simulink library "VLSGen"  (R2022b)
settings: Solver=VariableStepAuto  StartTime=0.0  StopTime=10.0  RelTol=1e-3
undefined symbols (not defined in the file or in its folder): Row, VLSConfig
libraries: TuneVar x3, TOP x2, FirGenericDeprecated x1, FeaturePath x1, FirGeneric x1
settings Model: Creator=ud1041536  LastModifiedBy=mt1047270
settings SolverCC: AlgebraicLoopSolver=TrustRegion
settings DataIOCC: ReturnWorkspaceOutputs=off
settings DebuggingCC: UnconnectedInputMsg=warning  UnconnectedOutputMsg=warning  UnconnectedLineMsg=warning  SFMachineParentedDataDiag=warning  ArithmeticOperatorsInVariantConditions=warning
settings ModelReferenceCC: EnableRefExpFcnMdlSchedulingChecks=on
settings SFSimCC: CustomCodeUndefinedFunction=UseInterfaceOnly

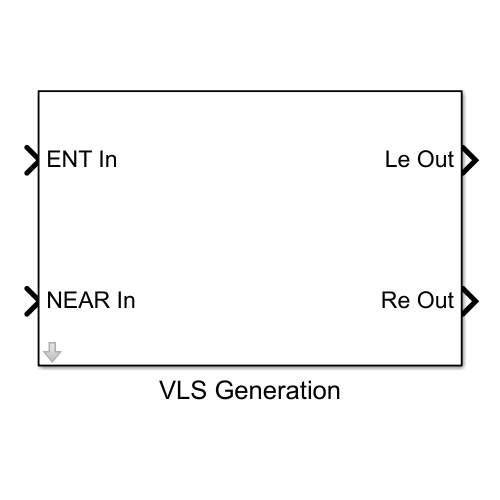
[thumbnail: Simulink's stored preview of the top-level diagram]
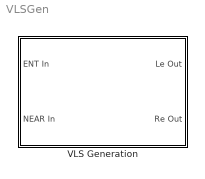
== system VLSGen ==
  VLS Generation : Subsystem  mask{configStruct=VLSConfig.VLSGenConfig, FeatureName=Generation}
      mask prompts: configStruct "Config struct name:"; FeatureName "Feature path name:"
      mask init:
      | % Get block parameters from configStruct
      | variantFIR = configStruct.variantFIR;
      | frameSize = configStruct.frameSize;
      | numFilters = configStruct.numFilters;
      | maxTotalFirLength = configStruct.maxTotalFirLength;
      | 
      | % Get block default values
      | firCoeffsDefault = configStruct.firCoeffsDefault;
      | firLengthsDefault = configStruct.firLengthsDefault;
      | 
      | % Set implementation type for FIR
      | % firBlockPath = MaskUtil.SubBlockName(gcbh, 'FIR');
      | % firBlockHandle = getSimulinkBlockHandle(firBlockPath);
      | % if -1 ~= firBlockHandle
      | %     set_param(firBlockHandle, 'variantSelect', variantFIR);
      | %     if variantFIR == 1 % Set two extras block params for Accel implementation
      | %         set_param(firBlockHandle, 'numIn', num2str(4));
      | %         set_param(firBlockHandle, 'frameSize', num2str(frameSize));
      | %     end
      | % end
      mask TypeOptions FeatureName: FeaturePath/FeatureName

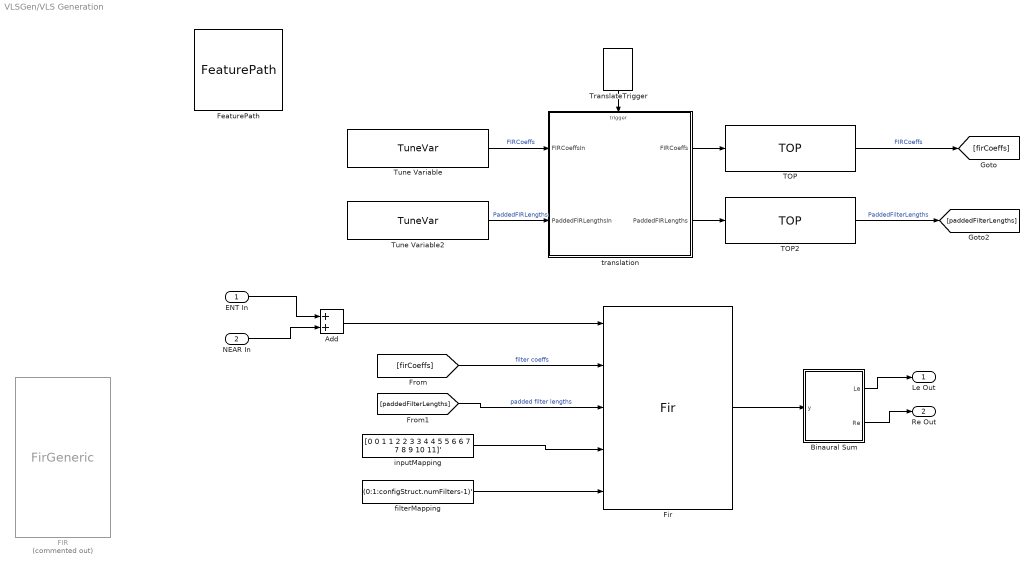
== system VLSGen/VLS Generation ==
  ENT In : Inport
  NEAR In : Inport  Port=2
  Add : Sum
  Binaural Sum : Subsystem
  FIR : FirGenericDeprecated/FirGeneric  Commented=on  Config=configStruct.Fir
  FeaturePath : FeaturePath/FeaturePath  FeatureName=Generation  IsGroup=off  GroupNumber=-1  IsModule=off  TriggerInit=[120 244 235 351]
      settings: SourceProductName=Bose Talaria
  Fir : FirGeneric/Fir  Config=configStruct.Fir
      settings: SourceProductName=Bose Blocklib
  TOP : TOP/TOP  TriggerInit=[815 370 985 430]  TopName=FIRCoeffs  DataTypeOut=single  BankNumber=1  PreOverlay=false  PostOverlay=false  Role=Automatic
      settings: SourceProductName=Bose Talaria
  TOP2 : TOP/TOP  TriggerInit=[815 465 985 525]  TopName=PaddedFilterLengths  DataTypeOut=uint32  BankNumber=0  PreOverlay=false  PostOverlay=false  Role=Automatic
      settings: SourceProductName=Bose Talaria
  TranslateTrigger : TuneVar/TranslateTrigger  TriggerInit=[656 270 694 325]
      settings: SourceProductName=Bose Talaria
  Tune Variable : TuneVar/TuneVar  TuneName=FIRCoeffs  SpecifyMaxSize=on  VariableDim=1 (Row)  MaxSize=[maxTotalFirLength 1]  TunabilityNumber=1  MinValue=[]  MaxValue=[]  TriggerInit=[320 375 505 425]  MaskValue=firCoeffsDefault
      settings: SourceProductName=Bose Talaria
  Tune Variable2 : TuneVar/TuneVar  TuneName=PaddedFIRLengths  SpecifyMaxSize=off  VariableDim=1 (Row)  MaxSize=[1 1]  TunabilityNumber=1  MinValue=[]  MaxValue=[]  TriggerInit=[320 470 505 520]  MaskValue=firLengthsDefault
      settings: SourceProductName=Bose Talaria
  filterMapping : Constant  Value=(0:1:configStruct.numFilters-1)'  VectorParams1D=off  OutDataTypeStr=uint32
  inputMapping : Constant  Value=[0 0 1 1 2 2 3 3 4 4 5 5 6 6 7 7 8 9 10 11]'  VectorParams1D=off  OutDataTypeStr=uint32
  translation : MATLAB Function  TreatAsAtomicUnit=on
  Le Out : Outport  VectorParamsAs1DForOutWhenUnconnected=off
  Re Out : Outport  Port=2  VectorParamsAs1DForOutWhenUnconnected=off
  wires:
  [firCoeffs] -> Fir/2  "filter coeffs"
  TOP/1 -> [firCoeffs]  "FIRCoeffs"
  filterMapping/1 -> Fir/5
  translation/1(FIRCoeffs) -> TOP/1
  TranslateTrigger/1 -> translation/Trigger
  Tune Variable/1 -> translation/1(FIRCoeffsIn)  "FIRCoeffs"
  inputMapping/1 -> Fir/4
  [paddedFilterLengths] -> Fir/3  "padded filter lengths"
  TOP2/1 -> [paddedFilterLengths]  "PaddedFilterLengths"
  translation/2(PaddedFIRLengths) -> TOP2/1
  NEAR In/1 -> Add/2
  Add/1 -> Fir/1
  ENT In/1 -> Add/1
  Fir/1 -> Binaural Sum/1(y)
  Binaural Sum/1(Le) -> Le Out/1
  Binaural Sum/2(Re) -> Re Out/1
  Tune Variable2/1 -> translation/2(PaddedFIRLengthsIn)  "PaddedFIRLengths"

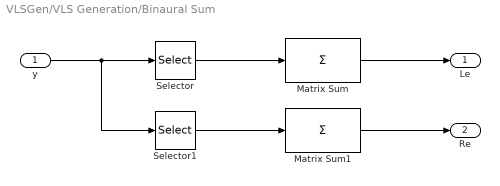
== system VLSGen/VLS Generation/Binaural Sum ==
  y : Inport
  Matrix Sum : Sum  Inputs=+  CollapseMode=Specified dimension  CollapseDim=2
  Matrix Sum1 : Sum  Inputs=+  CollapseMode=Specified dimension  CollapseDim=2
  Selector : Selector  NumberOfDimensions=2  InputPortWidth=3  IndexOptions=Select all,Index vector (dialog)  Indices=[1 3],configStruct.LeIdx  OutputSizes=1,1
  Selector1 : Selector  NumberOfDimensions=2  InputPortWidth=3  IndexOptions=Select all,Index vector (dialog)  Indices=[1 3],configStruct.ReIdx  OutputSizes=1,1
  Le : Outport  VectorParamsAs1DForOutWhenUnconnected=off
  Re : Outport  Port=2  VectorParamsAs1DForOutWhenUnconnected=off
  wires:
  Selector1/1 -> Matrix Sum1/1
  y/1 -> Selector/1, Selector1/1
  Selector/1 -> Matrix Sum/1
  Matrix Sum/1 -> Le/1
  Matrix Sum1/1 -> Re/1

== matlab function VLSGen/VLS Generation/translation ==
  data: FIRCoeffs output; FIRCoeffsIn input; PaddedFIRLengthsIn input; PaddedFIRLengths output
  events: trigger input FUNCTION_CALL_EVENT
function [FIRCoeffs, PaddedFIRLengths] = fcn(FIRCoeffsIn, PaddedFIRLengthsIn)

FIRCoeffs = FIRCoeffsIn.Value;
PaddedFIRLengths = PaddedFIRLengthsIn.Value;
